simulink model "sim_Ex4"  (R2022b)
settings: Solver=VariableStepAuto  StartTime=0.0  StopTime=10.0  FixedStep=1e-3  MaxStep=1e-4  RelTol=1e-4
libraries: spsVoltageMeasurementLib x2, spsParallelRLCBranchLib x1, spsControlledVoltageSourceLib x1, spsUniversalBridgeLib x1, eeRmsMeasurement x1, spsACVoltageSourceLib x1, spspowerguiLib x1
settings Model: Creator=MAAM  LastModifiedBy=MAAM

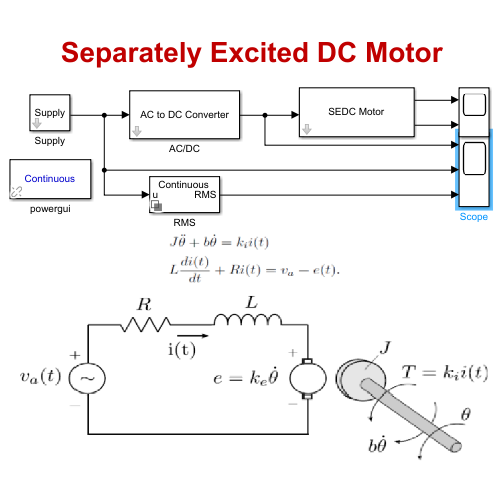
[thumbnail: Simulink's stored preview of the top-level diagram]
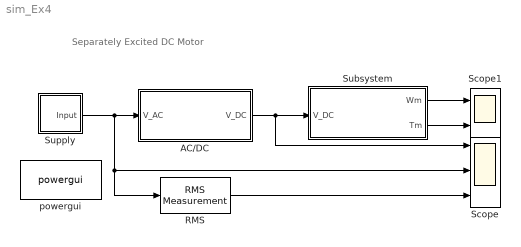
== system sim_Ex4 ==
  note: Separately Excited DC Motor
  AC/DC : Subsystem
      mask DialogControl DescGroupVar Prompt: AC-DC Converter
      mask Display: fprintf('AC to DC Converter');
  "RMS " : eeRmsMeasurement/RMS Measurement  LabelModeActiveChoice=Total  F=50  SpecifyHarmonics=off  K=[0 1 2]  Ts=0
      settings: LibrarySourceBlock=|
      | ee_sl_lib/Measurements/RMS
      | Measurement
  Scope : Scope  NumInputPorts=3
  Scope1 : Scope  NumInputPorts=2
  Subsystem : Subsystem  mask{TL=20, J=5, B=0.01, Ke=1.6, Ki=1.6, Ra=0.5, La=0.1}
      mask prompts: TL "Load Torque"; J "Rotor inertia (Kg.m^2) J"; B "Rotor friction (N.m.sec) B"; Ke "Back EMF constant (V.sec) Ke"; Ki "Torque constant (N.m/A) Ki"; Ra "Armature resistance (Ohm) Ra"; La "Armature inductance (H) La"
      mask Display: fprintf('SEDC Motor');
  Supply : Subsystem  mask{Vp=24*sqrt(2), F0=50}
      mask prompts: Vp "Peak Voltage V"; F0 "Frequency Hz"
      settings: PortSchema="{\"entries\":[{\"content\":{\"sides\":[{\"content\":{\"connectorIds\":[]},\"type\":\"ConnectorPlacement.EquallySpacedRectSide\",\"uuid\":\"46f37385-af1f-416a-a987-8572ff32bdb7\"},{\"content\":{\"connectorIds\":[],\"side\":\"RIGHT\"},\"type\":\"ConnectorPlacement.EquallySpacedRectSide\",\"uuid\":\"030bc9b7-c857-4180-ba8b-5482fb08a6e1\"},{\"content\":{\"connectorIds\":[],\"side\":\"TOP\"},\"type\":\"ConnectorPlacement.EquallySpacedRectSide\",\"uuid\":\"15ae90e8-d13e-4ac6-a01f-96cdc1009288\"},{\"content\":{\"connectorIds\":[\"Out1\"],\"side\":\"BOTTOM\"},\"type\":\"ConnectorPlacement.EquallySpacedRectSide\",\"uuid\":\"0e1449b7-f3b3-445e-a044-2164277e9aa2\"}]},\"type\":\"ConnectorPlacement.EquallySpacedConnector\",\"uuid\":\"b8180565-0155-4986-bb8e-4977057ae1f2\"}],\"packageUris\":[\"http://schema.mathworks.com/mf0/Connector/R2020b\"],\"version\":\"1.0\"}"
      mask Display: fprintf('Supply');
  powergui : spspowerguiLib/powergui  Priority=1  SimulationMode=Continuous  SampleTime=50e-6  frequency=60  Iterations=50  frequencyindice=50  Pbase=100e6  ErrMax=1e-4  UnitsV=kV  UnitsW=MW  buscounter=0  FunctionMessages=off  echomessages=off  EnableUseOfTLC=off  CurrentSourceSwitches=off  DisableSnubberDevices=off  DisableRonSwitches=off  DisableVfSwitches=off  DisplayEquations=off  AutomaticDiscreteSolvers=off  SolverType=Tustin/Backward Euler (TBE)  Interpol=off  ExternalGateDelay=off  methode=off  Ts=100  x0status=blocks  SPID=on  SwTol=0  HookPort=off  NonlinearTolerance=1e-4  nMaxIteration=100  ContinueOnMaxIteration=off  RestoreLinks=warning  ResistiveCurrentMeasurement=off  Frange=[0:2:500]  Ylog=off  Xlog=on  ShowGrid=off  save=off  variable=ZData  structure=0  ZoomFFT=off  StartTime=0.0  cycles=1  DisplayStyle=1  fundamental=60  FreqAxis=off  MaxFrequency=1000  frequencyindicesteady=1  RmsSteady=1  display=off
  wires:
  AC/DC/1(V_DC) -> Scope/1, Subsystem/1(V_DC)
  Subsystem/1(Wm) -> Scope1/1
  Supply/1(Input) -> "RMS "/1, Scope/2, AC/DC/1(V_AC)
  "RMS "/1 -> Scope/3
  Subsystem/2(Tm) -> Scope1/2

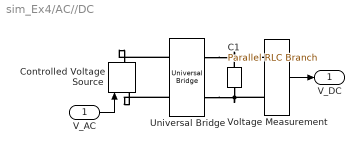
== system sim_Ex4/AC//DC ==
  V_AC : Inport
  C1 : spsParallelRLCBranchLib/Parallel RLC Branch  LConnTagsString=a  RConnTagsString=__new0  BranchType=C  Resistance=inf  Inductance=inf  SetiL0=off  InitialCurrent=0  Capacitance=1e-3  Setx0=off  InitialVoltage=0  Measurements=None
  Controlled Voltage Source : spsControlledVoltageSourceLib/Controlled Voltage Source  Initialize=on  Source_Type=AC  Amplitude=0  Phase=0  Frequency=0  Measurements=None
  Universal Bridge : spsUniversalBridgeLib/Universal Bridge  Arms=2  SnubberResistance=1e5  SnubberCapacitance=inf  Device=Diodes  Ron=1e-3  Lon=0  ForwardVoltages="[  0  0  ]"  ForwardVoltage=0  GTOparameters=[ 10e-6 , 20e-6 ]  IGBTparameters=[ 1e-6 , 2e-6 ]  Measurements=None  Measurements_2=None  converterType=Rectifier
  Voltage Measurement : spsVoltageMeasurementLib/Voltage Measurement  PhasorSimulation=off  OutputType=Complex  PSBequivalent=0
  V_DC : Outport
  wires:
  Voltage Measurement/1 -> V_DC/1
  V_AC/1 -> Controlled Voltage Source/1
  connections:
  Universal Bridge/LConn1 -- Controlled Voltage Source/RConn1
  Universal Bridge/LConn2 -- Controlled Voltage Source/LConn1
  C1/RConn1 -- Universal Bridge/RConn2 -- Voltage Measurement/LConn2
  Voltage Measurement/LConn1 -- Universal Bridge/RConn1 -- C1/LConn1

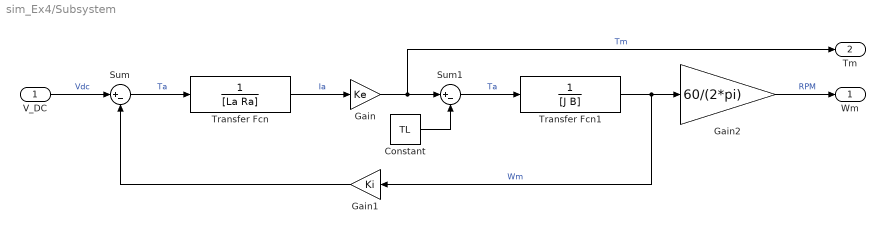
== system sim_Ex4/Subsystem ==
  V_DC : Inport
  Constant : Constant  Value=TL
  Gain : Gain  Gain=Ke
  Gain1 : Gain  Gain=Ki
  Gain2 : Gain  Gain=60/(2*pi)
  Sum : Sum  Inputs=|+-
  Sum1 : Sum  Inputs=|+-
  Transfer Fcn : TransferFcn  Denominator=[La Ra]
  Transfer Fcn1 : TransferFcn  Denominator=[J B]
  Wm : Outport
  Tm : Outport  Port=2
  wires:
  V_DC/1 -> Sum/1  "Vdc"
  Sum/1 -> Transfer Fcn/1  "Ta"
  Transfer Fcn/1 -> Gain/1  "Ia"
  Gain/1 -> Sum1/1, Tm/1  "Tm"
  Sum1/1 -> Transfer Fcn1/1  "Ta"
  Constant/1 -> Sum1/2
  Transfer Fcn1/1 -> Gain2/1, Gain1/1  "Wm"
  Gain2/1 -> Wm/1  "RPM"
  Gain1/1 -> Sum/2

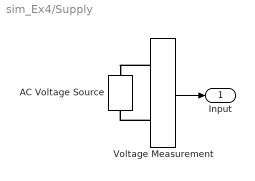
== system sim_Ex4/Supply ==
  AC Voltage Source : spsACVoltageSourceLib/AC Voltage Source  Amplitude=Vp  Phase=0  Frequency=F0  SampleTime=0  Measurements=None  BusType=swing  Pref=10e3  Qref=0  Qmin=-inf  Qmax=+inf
  Voltage Measurement : spsVoltageMeasurementLib/Voltage Measurement  PhasorSimulation=off  OutputType=Complex  PSBequivalent=0
  Input : Outport
  wires:
  Voltage Measurement/1 -> Input/1
  connections:
  Voltage Measurement/LConn1 -- AC Voltage Source/RConn1
  Voltage Measurement/LConn2 -- AC Voltage Source/LConn1
